simulink model "Simple_Pendulum_Simulation"  (R2023a)
settings: Solver=FixedStepAuto  StartTime=0.0  StopTime=10.0  FixedStep=1e-3  RelTol=1e-3
values from neighbouring files (symbols this model uses):
  g = 9.81    [Simple_Pendulum_Simulation(Automated_simulation_at_diff_values).m]
  L = runvalues(i)    [Simple_Pendulum_Simulation(Automated_simulation_at_diff_values).m]
settings Model: Creator=Mass  LastModifiedBy=Mass

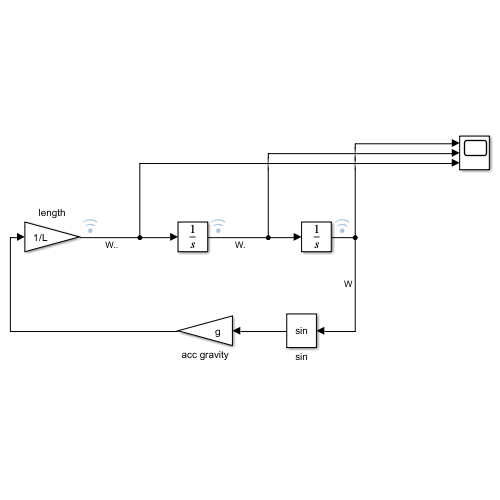
[thumbnail: Simulink's stored preview of the top-level diagram]
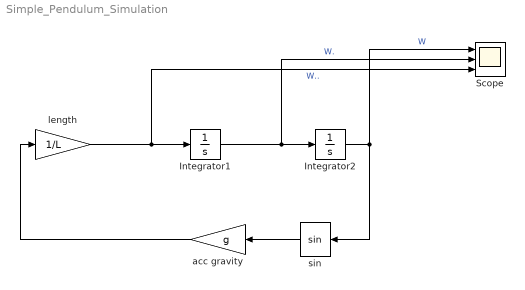
== system Simple_Pendulum_Simulation ==
  Integrator1 : Integrator  InitialCondition=1
  Integrator2 : Integrator
  Scope : Scope  NumInputPorts=3
  acc gravity : Gain  Gain=g
  length : Gain  Gain=1/L
  sin : Trigonometry
  wires:
  length/1 -> Scope/3, Integrator1/1  "W.."
  Integrator1/1 -> Scope/2, Integrator2/1  "W."
  Integrator2/1 -> sin/1, Scope/1  "W"
  sin/1 -> acc gravity/1
  acc gravity/1 -> length/1
